simulink model "sdrrSpectralAnalysisExample"  (R2020b)
settings: Solver=FixedStepDiscrete  StartTime=0.0  StopTime=inf  RelTol=1e-3  EnableMultiTasking=on
PostLoadFcn:
  | blk = 'sdrrSpectralAnalysisExample/Passband Spectrum';
  | cfg = get_param(blk,'ScopeConfiguration');
libraries: dspsigops x1, sdrrblksprivate x1, sdrrlib x1
CloseFcn:
  | clear blk cfg cf dialParam GetMaskObj maxCF minCF tune_cmd;
settings Model: Creator=The MathWorks, Inc.  LastModifiedBy=trevor
settings DataIOCC: LimitDataPoints=on  SaveFormat=Array  SaveOutput=off  SignalLogging=off  DSMLogging=off  SaveTime=off  ReturnWorkspaceOutputs=off
settings OptimizationCC: ExpressionDepthLimit=2147483647  LifeSpan=inf
settings DebuggingCC: UnderspecifiedInitializationDetection=Classic  MergeDetectMultiDrivingBlocksExec=none  SolverPrmCheckMsg=warning  ParameterPrecisionLossMsg=none  FcnCallInpInsideContextMsg=warning  AllowSymbolicDim=off  StateNameClashWarn=warning  SFUnexpectedBacktrackingDiag=warning  SFNoUnconditionalDefaultTransitionDiag=warning  SFExecutionAtInitializationDiag=none  ArithmeticOperatorsInVariantConditions=warning
settings HardwareCC: ProdBitPerPointer=32  ProdBitPerSizeT=32  ProdBitPerPtrDiffT=32  ProdLargestAtomicFloat=None  ProdIntDivRoundTo=Undefined  ProdEndianess=Unspecified  ProdWordSize=32  ProdHWDeviceType=32-bit Generic  TargetBitPerLong=64  TargetBitPerPointer=64  TargetBitPerSizeT=64  TargetBitPerPtrDiffT=64  TargetLongLongMode=on  TargetIntDivRoundTo=Zero  TargetEndianess=LittleEndian  TargetWordSize=64  TargetHWDeviceType=Generic->MATLAB Host Computer  ProdEqTarget=off
settings ModelReferenceCC: PropagateSignalLabelsOutOfModel=off
settings SFSimCC: SimUseLocalCustomCode=off  CustomCodeUndefinedFunction=UseInterfaceOnly
settings RTWCC: RTWUseLocalCustomCode=off
settings RTWCC: CustomSourceCode=|
  | #include<stdio.h>
  | #include<stdlib.h>
settings CodeAppCC: StateflowObjectComments=on
settings GRTTargetCC: TargetLangStandard=C89/C90 (ANSI)  CombineOutputUpdateFcns=off  GRTInterface=on
settings ConfigComp: CovMetricSettings=dw  CovSaveCumulativeToWorkspaceVar=on  CovSaveSingleToWorkspaceVar=on  CovExternalEMLEnable=off  CovSFcnEnable=off

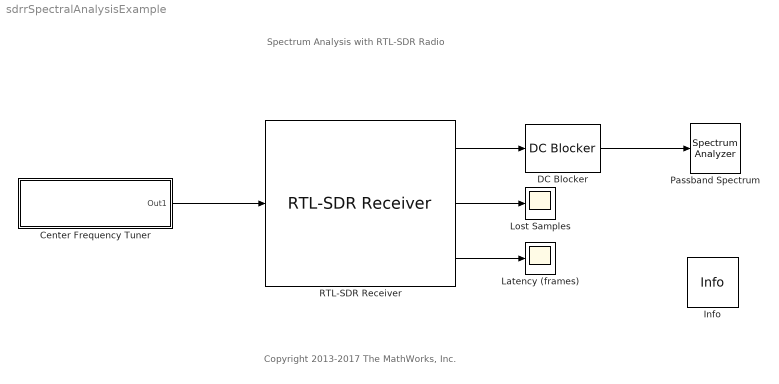
== system sdrrSpectralAnalysisExample ==
  note: Spectrum Analysis
      | with RTL-SDR Radio
  note: Copyright 2013-2017 The MathWorks, Inc.
  Center Frequency Tuner : Subsystem  mask{CenterFrequency=919.100, MinCenterFrequency=910, MaxCenterFrequency=920}
      mask prompts: CenterFrequency "Center Frequency (MHz)"; MinCenterFrequency "Min Center Frequency (MHZ)"; MaxCenterFrequency "Max Center Frequency (MHz)"
      mask Callback CenterFrequency:
      | % Get the center frequency value from the center frequency tuner
      | cf = str2num(get_param(gcb,'CenterFrequency'));
      | if isempty(cf)
      |     % Default Value
      |     cf = 102.5;
      | end
      | cf = cf.*1e6;
      | % Tune command used to set the Frequency offset on the spectrum analyzer
      | tune_cmd = ['cfg.FrequencyOffset = ''' num2str(cf) ''';'];
      | % Evaluate the tuning command in the base workspace
      | evalin('base',tune_cmd);
      mask Callback MinCenterFrequency:
      | GetMaskObj = Simulink.Mask.get(gcb);
      | dialParam = GetMaskObj.getParameter('CenterFrequency');
      | minCF = get_param(gcb,'MinCenterFrequency');
      | maxCF = get_param(gcb,'MaxCenterFrequency');
      | if isempty(minCF)
      |     minCF = 87.7;
      | end
      | if isempty(maxCF)
      |    macCF = 107.9;
      | end
      | 
      | if ~isempty(minCF) && ~isempty(maxCF)
      |  try
      |     dialParam.Range = [str2num(minCF),str2num(maxCF)];
      |  catch
      |  end
      | end
      mask Callback MaxCenterFrequency:
      | GetMaskObj = Simulink.Mask.get(gcb);
      | dialParam = GetMaskObj.getParameter('CenterFrequency');
      | minCF = get_param(gcb,'MinCenterFrequency');
      | maxCF = get_param(gcb,'MaxCenterFrequency');
      | if isempty(minCF)
      |     minCF = 87.7;
      | end
      | if isempty(maxCF)
      |    macCF = 107.9;
      | end
      | 
      | if ~isempty(minCF) && ~isempty(maxCF)
      |  try
      |     dialParam.Range = [str2num(minCF),str2num(maxCF)];
      |  catch
      |  end
      | end
      mask DialogControl CenterFrequencyContainer Prompt: SDR Center Frequency (MHz)
      mask DialogControl FrequencyRangeContainer Prompt: Frequency Range (MHz)
      mask Display: fprintf('Center Frequency = %3.1f MHz',CenterFrequency);
  DC Blocker : dspsigops/DC Blocker  Algorithm=Subtract mean  NormalizedBandwidth=0.001  Length=50  Order=6  SimulateUsing=Code generation
      settings: SourceProductName=DSP System Toolbox
  Info : sdrrblksprivate/Info  SystemSampleTime=-1  VariantActivationTime=update diagram  Latency=0  AutoFrameSizeCalculation=off
      settings: SourceProductBaseCode=RTLSDR
  Latency (frames) : Scope
  Lost Samples : Scope
  Passband Spectrum : SpectrumAnalyzer
  RTL-SDR Receiver : sdrrlib/RTL-SDR Receiver  IPAddress=0  CenterFrequencySource=Input port  CenterFrequency=102.5e6  GainSource=AGC  Gain=0  ADCRate=2e6  FrequencyCorrection=0  LostSamplesOutputPort=on  LatencyOutputPort=on  OutputDataType=double  FrameLength=256*20  EnableBurstMode=off  NumFramesInBurst=20  sobjType=sdrr.internal.SDRRTLReceiverSL  dataUDPPort=-1  ctrlUDPPort=-1  subDeviceList=nosubdev  sdrBlockType=SDRBlockTypeSLT.SDRRxBlock  requester=UNUSED_BY_SFCN  sdrExecutionMode=SDRExecutionModeSLT.ExecModeHW  BypassUserLogic=off  DecimatorSelect=DDC decimator  SourceSelect=Sine generator  SineAmplitude=16000  EnableInternalClock=off  BypassIQBalance=off  IFBandwidth=40e6  ADCRateSource=Dialog  IntermediateFrequency=0  DecimationFactorSource=Dialog  DecimationFactor=512  RFFrequencyIsTunable=logical(1)  SampleTime=(256*20)/(2e6)  IFBandwidthSource=Dialog  SineFrequency=30000  BypassDCBlockingFilter=off  IntermediateFrequencySource=Dialog  IQBalanceCoefficients=64  SkipAllHardwareResetAndInitialization=off  EnableIQCalibrationTable=on  CacheIQCalibrationTable=off  EnableOffsetTuning=off  EnableRTLAGC=off  EnableTestMode=off  EnableTunerAGC=on  FrequencyCorrectionSource=Dialog  NumMLBuffers=128  NumUSBBuffers=16  RTLCrystalFrequency=28800000  TunerCrystalFrequency=28800000
      settings: SourceProductName=Communications Toolbox Support Package for RTL-SDR Radio
  wires:
  RTL-SDR Receiver/1 -> DC Blocker/1
  DC Blocker/1 -> Passband Spectrum/1
  RTL-SDR Receiver/2 -> Lost Samples/1
  RTL-SDR Receiver/3 -> Latency (frames)/1
  Center Frequency Tuner/1(Out1) -> RTL-SDR Receiver/1

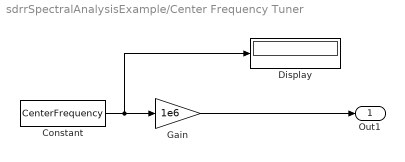
== system sdrrSpectralAnalysisExample/Center Frequency Tuner ==
  Constant : Constant  Value=CenterFrequency  SampleTime=-1
  Display : Display
  Gain : Gain  Gain=1e6
  Out1 : Outport  VectorParamsAs1DForOutWhenUnconnected=off
  wires:
  Constant/1 -> Display/1, Gain/1
  Gain/1 -> Out1/1
